simulink model "N_indiv"  (R2022a)
settings: Solver=FixedStepDiscrete  StartTime=0.0  StopTime=86000  FixedStep=SimulationStep  RelTol=1e-3
undefined symbols (not defined in the file or in its folder): Bid_baisse, Bid_hausse, SimulationStep
settings Model: PacingRate=1000  Creator=a.dehghan  LastModifiedBy=a.dehghan

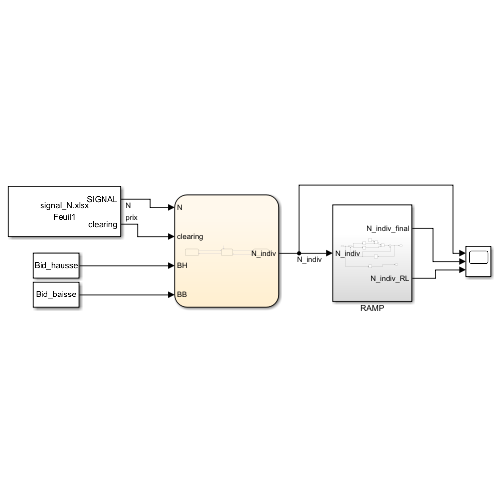
[thumbnail: Simulink's stored preview of the top-level diagram]
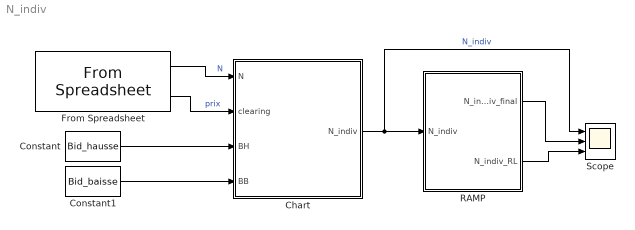
== system N_indiv ==
  Chart : Stateflow chart  TreatAsAtomicUnit=on
  Constant : Constant  Value=Bid_hausse
  Constant1 : Constant  Value=Bid_baisse
  From Spreadsheet : FromSpreadsheet  FileName=signal_N.xlsx  SheetName=Feuil1
  RAMP : Subsystem
  Scope : Scope  NumInputPorts=3
  wires:
  Chart/1(N_indiv) -> Scope/1, RAMP/1(N_indiv)  "N_indiv"
  Constant1/1 -> Chart/4(BB)
  Constant/1 -> Chart/3(BH)
  From Spreadsheet/1 -> Chart/1(N)  "N"
  From Spreadsheet/2 -> Chart/2(clearing)  "prix"
  RAMP/1(N_indiv_final) -> Scope/2
  RAMP/2(N_indiv_RL) -> Scope/3

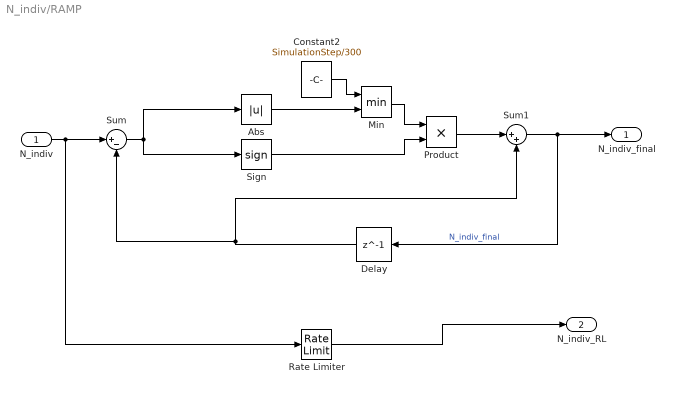
== system N_indiv/RAMP ==
  N_indiv : Inport
  Abs : Abs  SaturateOnIntegerOverflow=off
  Constant2 : Constant  Value=SimulationStep/300
  Delay : Delay  DelayLength=1
  Min : MinMax  Inputs=2
  Product : Product
  Rate Limiter : RateLimiter  RisingSlewLimit=1/300  FallingSlewLimit=-1/300  SampleTimeMode=inherited  LinearizeAsGain=off
  Sign : Signum
  Sum : Sum  Inputs=|+-
  Sum1 : Sum  Inputs=|++
  N_indiv_final : Outport
  N_indiv_RL : Outport  Port=2
  wires:
  Sum/1 -> Sign/1, Abs/1
  Delay/1 -> Sum1/2, Sum/2
  Product/1 -> Sum1/1
  Min/1 -> Product/1
  Sum1/1 -> Delay/1, N_indiv_final/1  "N_indiv_final"
  Sign/1 -> Product/2
  Abs/1 -> Min/2
  Constant2/1 -> Min/1
  N_indiv/1 -> Rate Limiter/1, Sum/1
  Rate Limiter/1 -> N_indiv_RL/1

== stateflow chart N_indiv/Chart ==
  state Baisse
    en : clearing <= BB;
    N_indiv = -1;
  state N_0
    en : N_indiv = 0;
  state Hausse
    en :  clearing >= BH;
    N_indiv = 1;
  (default) -> N_0
  Baisse -> N_0 : [N == 0]
  N_0 -> Hausse [order 1] : [N > 0 ]
  N_0 -> Baisse [order 2] : [N < 0]
  Hausse -> N_0 : [N == 0]
  data: N input; clearing input; BH input; BB input; N_indiv output
